simulink library "acc"  (R2021b)
settings: Solver=VariableStepAuto  StartTime=0.0  StopTime=10.0  RelTol=1e-3
undefined symbols (not defined in the file or in its folder): AACC_EHPSSpdCtrlMode_X_enum, AACC_EHPSSpdCtrlMode_Y_rad, ENUM__SASCALED_CALED, ENUM_BRAKEPEDAL_RELEASED, ENUM_CACENABLESTS_RUN, ENUM_DCDCENABLESTS_RUN, ENUM_EHPSCTRLMODE_FULLPWR, ENUM_EHPSCTRLMODE_NORMAL, ENUM_EHPSCTRLMODE_STEP1, ENUM_EHPSCTRLMODE_ZERO, ENUM_EHPSENABLESTS_INITIAL, ENUM_EHPSENABLESTS_READY, ENUM_EHPSENABLESTS_RUN, ENUM_PMMMODE_DRIVE, ENUM_PMMMODE_POWERUP, ENUM_TARGETGEAR_NEUTRAL, FALSE, KACC_AirPressInvalid_kpa, KACC_CACEnableFailTime_s, KACC_CACOverrunRcvTime_s, KACC_CACOverrunTime_min, KACC_CACOverTempDelayTime_s, KACC_CACOverTempRcv_s, KACC_CACPresLow_kPa, KACC_CACPressureSWRev_flg, KACC_CACPresWarn_kPa, KACC_CACPresWarn_ovrdflg_flg, KACC_CACPresWarn_ovrdval_flg, KACC_CACStopTime_s, KACC_CACTemp_C, KACC_CACTempRev_C, KACC_CACTempStop_C, KACC_CACTempWarn_C, KACC_CACValid_flg, KACC_CP2VAutoTracH_enum, KACC_CP2VDamStiffReqFA_pct, KACC_CP2VDamStiffReqLA_pct, KACC_CP2VDamStiffReqRA_pct, KACC_CP2VKneeCtrlMReq_enum, KACC_CP2VKneeReqFA_enum, KACC_CP2VKneeReqRA_enum, KACC_CP2VKneeReqRSide_enum, KACC_CP2VLA1PosCmd_enum, KACC_CP2VLA2PosCmd_enum, KACC_CP2VLvCtrlModeReq_enum, KACC_CP2VNLvReqFA_enum, KACC_CP2VNLvReqRA_enum, KACC_DCDCErrLvHoldtime_s, KACC_DTCACCReset_flg, KACC_DTCCACOverrun_cnt, KACC_EACErrLvHoldtime_s, KACC_ECASKneeSideSW_flg, KACC_EcasSw1Down_flg, KACC_EcasSw1Up_flg, KACC_EcasSw2M2_flg, KACC_EcasSw2Stop_flg, KACC_EcasSw3Knee_flg, KACC_EcasSw3M1_flg, KACC_EcasSwDebounceTime_s, KACC_ECASSwitch_flg ... (+30)
libraries: hcu_lib x20, simulink x3
(part 1 of 3)
settings Model: Creator=zack  LastModifiedBy=zack

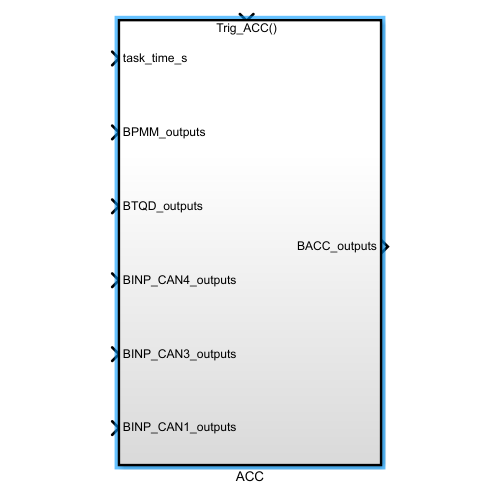
[thumbnail: Simulink's stored preview of the top-level diagram]
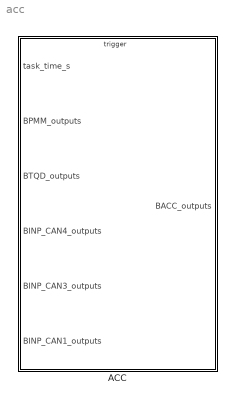
== system acc ==
  ACC : Subsystem  TreatAsAtomicUnit=on
      settings: RTWSystemCode=Nonreusable function  RTWFcnNameOpts=Use subsystem name  RTWFileNameOpts=Use subsystem name

== system acc/ACC ==
  task_time_s : Inport
  BPMM_outputs : Inport  Port=2  OutDataTypeStr=Bus: BPMM_outputs
  BTQD_outputs : Inport  Port=3  OutDataTypeStr=Bus: BTQD_outputs
  BINP_CAN4_outputs : Inport  Port=4  OutDataTypeStr=Bus: BINP_CAN4_outputs
  BINP_CAN3_outputs : Inport  Port=5  OutDataTypeStr=Bus: BINP_CAN3_outputs
  BINP_CAN1_outputs : Inport  Port=6  OutDataTypeStr=Bus: BINP_CAN1_outputs
  Trig_ACC : TriggerPort  TriggerType=function-call  VariantControl=(inherit)
  Input_Convert : Subsystem
  Main : Subsystem
  Model Info1 : hcu_lib/Model Info1  BlockCM=None  Frame=on  DisplayStringWithTags=|  HorizontalTextAlignment=Left  LeftAlignmentValue=0.02  SourceBlockDiagram=hcu_lib  TagMaxNumber=20
      | Model Version        : %<ModelVersion>
      | Creator                   : %<Creator>
      | Last Modified By    : %<LastModifiedBy>
      settings: SourceProductName=HCU Relative Block Library
  OutpConvert : Subsystem
  SCP_In : Subsystem
  SCP_Out : Subsystem
  BACC_outputs : Outport  OutDataTypeStr=Bus: BACC_outputs  VectorParamsAs1DForOutWhenUnconnected=off
  wires:
  task_time_s/1 -> SCP_In/1(task_time_s)
  BINP_CAN4_outputs/1 -> SCP_In/2(BINP_CAN4_outputs)
  BINP_CAN3_outputs/1 -> SCP_In/3(BINP_CAN3_outputs)
  BINP_CAN1_outputs/1 -> SCP_In/4(BINP_CAN1_outputs)
  BTQD_outputs/1 -> SCP_In/5(BTQD_outputs)
  BPMM_outputs/1 -> SCP_In/6(BPMM_outputs)
  SCP_In/1(BSCP_In_outputs) -> [BSCP_In_outputs]
  [BSCP_In_outputs] -> Input_Convert/1(BSCP_In_outputs)
  Input_Convert/1(BInpConvert_outputs) -> [BInpConvert_outputs]
  [BInpConvert_outputs] -> Main/2(BInpConvert_outputs)
  [BSCP_In_outputs] -> Main/1(BSCP_In_outputs)
  Main/1(BMain_outputs) -> [BMain_outputs]
  [BMain_outputs] -> Input_Convert/2(BMain_outputs)
  [BInpConvert_outputs] -> OutpConvert/2(BInpConvert_outputs)
  [BMain_outputs] -> OutpConvert/3(BMain_outputs)
  [BSCP_In_outputs] -> OutpConvert/1(BSCP_In_outputs)
  OutpConvert/1(BOutpConvert_outputs) -> [BOutpConvert_outputs]
  [BInpConvert_outputs] -> SCP_Out/1(BInpConvert_outputs)
  [BMain_outputs] -> SCP_Out/2(BMain_outputs)
  [BOutpConvert_outputs] -> SCP_Out/3(BOutpConvert_outputs)
  SCP_Out/1(BACC_outputs) -> BACC_outputs/1

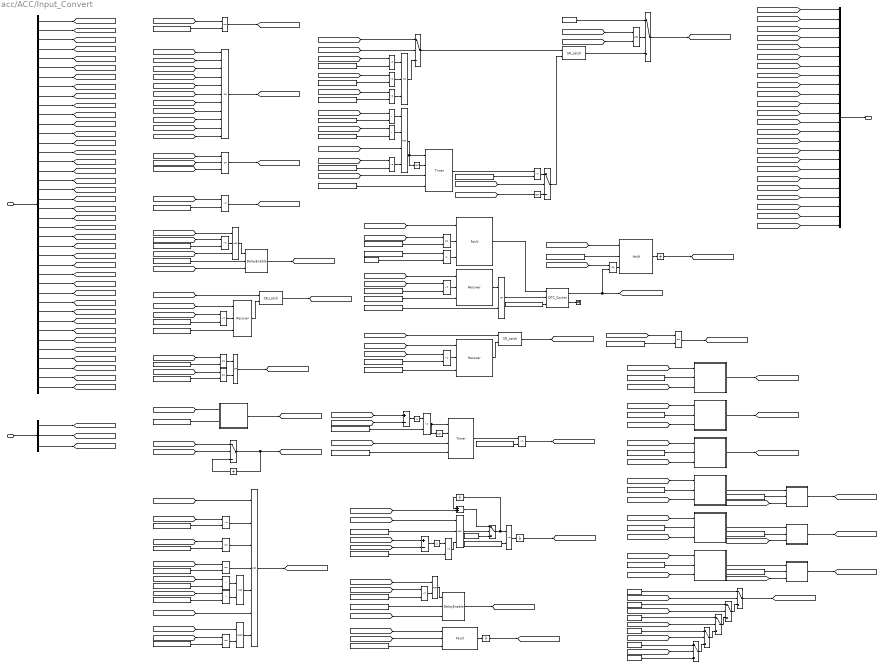
== system acc/ACC/Input_Convert ==
  note: ECAS Demand Determination From Pin
  note: EHPS Force Stop Detection
  note: EHPS Motor Speed Demand TimeOut Detection
  note: EHPS Disable Judgement
  note: Steering Wheel Moving Detection
  note: Steering Angle has been calabrated flag
  note: EHPS Error Hold Disable Judgment
  note: EHPS Cooling Mode Judgment
  note: Brake Pedal Released Flag
  note: EAC Pressure Sensor DDM
  note: EAC Pressure Switch DDM
  note: EAC Over Temperature Judgment
  note: EAC Pressure Low Judgment
  note: EAC Running Fail Judgment
  note: EAC Forece Stop Judgment
  note: EAC Error Hold Disable Judgment
  BSCP_In_outputs : Inport
  BMain_outputs : Inport  Port=2
  " EcasSw1Down Debounce" : Subsystem
  " EcasSw1Up Debounce" : Subsystem
  " EcasSw2Stop Debounce" : Subsystem
  AND : Logic  Inputs=4  AllPortsSameDT=off  OutDataTypeStr=boolean
  AND1 : Logic  AllPortsSameDT=off  OutDataTypeStr=boolean
  AND2 : Logic  AllPortsSameDT=off  OutDataTypeStr=boolean
  AND3 : Logic  Inputs=3  AllPortsSameDT=off  OutDataTypeStr=boolean
  AND5 : Logic  Operator=NAND  AllPortsSameDT=off  OutDataTypeStr=boolean
  Abs : Abs
  Abs1 : Abs
  Add : Sum  Inputs=+-
  Add1 : Sum  Inputs=+-
  Add2 : Sum
  Bus Creator : BusCreator  Inputs=24
  Bus Selector : BusSelector  OutputSignals=VINP_EBSBrakeSw_enum,VDMM_DTCFCShortBatt_flg,VDMM_DTCPCShortBatt_flg,VDMM_DTCRCShortBatt_flg,VDMM_DTCFCOpenGND_flg,VDMM_DTCPCOpenGND_flg,VDMM_DTCRCOpenGND_flg,VDMM_DTCFCStuckHigh_flg,VDMM_DTCRCStuckHigh_flg,VDMM_DTCFCStuckLow_flg,VDMM_DTCPCStuckLow_flg,VDMM_DTCRCStuckLow_flg,VDMM_DTCAirSwError_flg,VDMM_DTCAirSwStuckClose_flg,VDMM_DTCAirSwStuckOpen_flg,VINP_CACTemp_C,VINP_FDCCHASSISVCUEACPressSta_flg,VINP_AirPressureRC1_kPa,VINP_AirPressureFC2_kPa,VINP_AirPressurePC3_kPa,task_time_s,VINP_EACEnSta_enum,VPMM_EACEnableCompleted_flg,VDMM_DTCEACErrLv_flg,VPMM_SysPowerMode_enum,VDMM_DTCEHPSErrLv_flg,VINP_EHPSEnSta_enum,VINP_SASCaled_enum,VINP_StrWhlAng_rad,VINP_ParkBrakeSW_enum,VTQD_VCUVehSpd_kph,VINP_TransReqGear_enum,VDMM_DTCEHPSRlyNoFB_flg,VINP_EHPSMotorSpdSta_rpm,VINP_EcasSw1Up_flg,VINP_EcasSw1Down_flg,VINP_EcasSw2Stop_flg,VINP_EcasSw2M2_flg,VINP_EcasSw3M1_flg,VINP_EcasSw3Knee_flg
  Bus Selector1 : BusSelector  OutputSignals=VACC_CACEnableDem_flg,VACC_InitEHPSEnDem_flg,VACC_EHPSMotorDemSpd_rpm
  Constant : Constant  Value=ENUM_BRAKEPEDAL_RELEASED
  Constant1 : Constant  Value=KACC_CACPresLow_kPa
  Constant10 : Constant  Value=KACC_CACPresWarn_kPa
  Constant11 : Constant  Value=MIN2SEC
  Constant12 : Constant  Value=KACC_DTCCACOverrun_cnt
  Constant13 : Constant  Value=KACC_CACOverrunRcvTime_s
  Constant131 : Constant  Value=KACC_SpeedOverEHPSEnDemend_kph
  Constant{14..15,17,22} (4 alike) : Constant  Value=ENUM_CACENABLESTS_RUN
  Constant16 : Constant  Value=KACC_DTCACCReset_flg
  Constant18 : Constant  Value=KACC_CACEnableFailTime_s
  Constant19 : Constant  Value=KACC_CACOverrunTime_min
  Constant2 : Constant  Value=TRUE
  Constant20 : Constant  Value=KACC_CACStopTime_s
  Constant21 : Constant  Value=KACC_EACErrLvHoldtime_s
  Constant23 : Constant  Value=ENUM_PMMMODE_DRIVE  SampleTime=-1
  Constant24 : Constant  Value=ENUM_PMMMODE_POWERUP  SampleTime=-1
  Constant25 : Constant  Value=KACC_EHPSErrLvHoldtime_s
  Constant26 : Constant  Value=ENUM_EHPSENABLESTS_RUN
  Constant27 : Constant  Value=ENUM__SASCALED_CALED
  Constant28 : Constant  Value=KACC_StrWhlAngSampleTime_s
  Constant29 : Constant  Value=KACC_EHPSDisStrWhlDiv_rad
  Constant3 : Constant  Value=KACC_CACPresWarn_kPa
  Constant30 : Constant  Value=KACC_StrWhlNotMovingTime_s  OutDataTypeStr=single
  Constant31 : Constant  Value=KACC_StrWhlNotMovingTime_s  OutDataTypeStr=single
  Constant32 : Constant  Value=KACC_EHPSDisStrWhlHi_rad
  Constant33 : Constant  Value=KACC_EHPSDisStrWhlLo_rad
  Constant34 : Constant  Value=ENUM_PMMMODE_DRIVE
  Constant35 : Constant  Value=ENUM_TARGETGEAR_NEUTRAL
  Constant36 : Constant  Value=ENUM__SASCALED_CALED
  Constant37 : Constant  Value=KACC_EHPSCtrlModeStep2_flg
  Constant38 : Constant  Value=KACC_EHPSSpdDiv_rpm
  Constant39 : Constant  Value=ENUM_EHPSENABLESTS_RUN
  Constant4 : Constant  Value=KACC_CACPresWarn_kPa
  Constant40 : Constant  Value=KACC_EHPSEnableFailTime_s
  Constant41 : Constant  Value=KACC_EHPSStopTime_s
  Constant{42..47} (6 alike) : Constant  Value=KACC_EcasSwDebounceTime_s
  Constant48 : Constant  Value=KACC_EcasSwTrigHoldTime_s
  Constant49 : Constant  Value=KACC_EcasSwTrigHoldTime_s
  Constant5 : Constant  Value=KACC_SwitchFailSensorRef_kpa
  Constant50 : Constant  Value=KACC_EcasSwTrigHoldTime_s
  Constant51 : Constant  Value=uint8(0)
  Constant52 : Constant  Value=uint8(7)
  Constant53 : Constant  Value=uint8(2)
  Constant54 : Constant  Value=uint8(6)
  Constant55 : Constant  Value=uint8(1)
  Constant56 : Constant  Value=uint8(8)
  Constant6 : Constant  Value=KACC_SwitchFailSensorRef_kpa
  Constant62 : Constant  Value=ZERO_FLOAT
  Constant63 : Constant  Value=KACC_EHPSSpdDemTimeout_s
  Constant7 : Constant  Value=KACC_SwitchFailSensorRefRcv_s
  Constant8 : Constant  Value=KACC_SwitchFailSensorRefRcv_s
  Constant9 : Constant  Value=KACC_CACTempStop_C
  DTC_Couter : hcu_lib/Basic_Blocks/DTC_Couter
      settings: SourceProductName=HCU Relative Block Library
  DelayEnable : hcu_lib/Basic_Blocks/DelayEnable
      settings: SourceProductName=HCU Relative Block Library
  DelayEnable1 : hcu_lib/Basic_Blocks/DelayEnable
      settings: SourceProductName=HCU Relative Block Library
  EcasSw2M2 Debounce : Subsystem
  EcasSw3Knee Debounce : Subsystem
  EcasSw3M1 Debounce : Subsystem
  Equal{,1..2,5,9} (5 alike) : RelationalOperator  Operator===  OutDataTypeStr=boolean  RndMeth=Simplest
  Equal3 : RelationalOperator  Operator=<  OutDataTypeStr=boolean  RndMeth=Simplest
  Equal4 : RelationalOperator  Operator=<=  OutDataTypeStr=boolean  RndMeth=Simplest
  Equal6 : RelationalOperator  Operator=>  OutDataTypeStr=boolean  RndMeth=Simplest
  Fault : hcu_lib/Basic_Blocks/Fault  SystemSampleTime=-1  VariantActivationTime=update diagram  Latency=0  AutoFrameSizeCalculation=off
      settings: SourceProductName=HCU Relative Block Library
  Fault1 : hcu_lib/Basic_Blocks/Fault  SystemSampleTime=-1  VariantActivationTime=update diagram  Latency=0  AutoFrameSizeCalculation=off
      settings: SourceProductName=HCU Relative Block Library
  Hold1 : hcu_lib/Basic_Blocks/Hold  SystemSampleTime=-1  VariantActivationTime=update diagram  Latency=0  AutoFrameSizeCalculation=off
      settings: SourceProductName=HCU Relative Block Library
  Logical Operator : Logic  Operator=OR  AllPortsSameDT=off  OutDataTypeStr=boolean
  Logical Operator1 : Logic  AllPortsSameDT=off  OutDataTypeStr=boolean
  Logical Operator10 : Logic  Operator=OR  Inputs=3  AllPortsSameDT=off  OutDataTypeStr=boolean
  Logical Operator4 : Logic  Inputs=7  AllPortsSameDT=off  OutDataTypeStr=boolean
  Logical Operator5 : Logic  Inputs=3  AllPortsSameDT=off  OutDataTypeStr=boolean
  Logical Operator6 : Logic  Operator=OR  AllPortsSameDT=off  OutDataTypeStr=boolean
  NOT : Logic  Operator=NOT  AllPortsSameDT=off  OutDataTypeStr=boolean
  NOT1 : Logic  Operator=NOT  AllPortsSameDT=off  OutDataTypeStr=boolean
  NOT4 : Logic  Operator=NOT  AllPortsSameDT=off  OutDataTypeStr=boolean
  OR : Logic  Operator=OR  Inputs=11  AllPortsSameDT=off  OutDataTypeStr=boolean
  OR1 : Logic  Operator=OR  Inputs=3  AllPortsSameDT=off  OutDataTypeStr=boolean
  OR2 : Logic  Operator=OR  AllPortsSameDT=off  OutDataTypeStr=boolean
  Product : Product
  Recover : hcu_lib/Basic_Blocks/Recover  SystemSampleTime=-1  VariantActivationTime=update diagram  Latency=0  AutoFrameSizeCalculation=off
      settings: SourceProductName=HCU Relative Block Library
  Recover1 : hcu_lib/Basic_Blocks/Recover  SystemSampleTime=-1  VariantActivationTime=update diagram  Latency=0  AutoFrameSizeCalculation=off
      settings: SourceProductName=HCU Relative Block Library
  Recover2 : hcu_lib/Basic_Blocks/Recover  SystemSampleTime=-1  VariantActivationTime=update diagram  Latency=0  AutoFrameSizeCalculation=off
      settings: SourceProductName=HCU Relative Block Library
  Relational Operator{,8,11..12,16,18} (6 alike) : RelationalOperator  OutDataTypeStr=boolean  RndMeth=Simplest
  Relational Operator{1..2,9,15,19} (5 alike) : RelationalOperator  Operator=~=  OutDataTypeStr=boolean  RndMeth=Simplest
  Relational Operator10 : RelationalOperator  Operator===  OutDataTypeStr=boolean  RndMeth=Nearest
  Relational Operator{6..7,13,17} (4 alike) : RelationalOperator  Operator=<=  OutDataTypeStr=boolean  RndMeth=Simplest
  Relational Operator14 : RelationalOperator  Operator===  OutDataTypeStr=boolean  RndMeth=Nearest
  Relational Operator3 : RelationalOperator  Operator=>  OutDataTypeStr=boolean  RndMeth=Simplest
  Relational Operator4 : RelationalOperator  Operator===  OutDataTypeStr=boolean  RndMeth=Simplest
  Relational Operator5 : RelationalOperator  Operator=>  OutDataTypeStr=boolean  RndMeth=Simplest
  SR_Latch : hcu_lib/Basic_Blocks/SR_Latch
      settings: SourceProductName=HCU Relative Block Library
  SR_Latch1 : hcu_lib/Basic_Blocks/SR_Latch
      settings: SourceProductName=HCU Relative Block Library
  SR_Latch2 : hcu_lib/Basic_Blocks/SR_Latch
      settings: SourceProductName=HCU Relative Block Library
  Switch{,1..9} (10 alike) : Switch  Criteria=u2 ~= 0
      settings: AttributesFormatString=%<Criteria>
  Switch hold : Subsystem
  Switch hold1 : Subsystem
  Switch hold3 : Subsystem
  Terminator1 : Terminator
  Timer : hcu_lib/Basic_Blocks/Timer
      settings: SourceProductName=HCU Relative Block Library
  Timer1 : hcu_lib/Basic_Blocks/Timer
      settings: SourceProductName=HCU Relative Block Library
  Trigger : Subsystem  AncestorBlock=hcu_lib/Basic_Blocks/Fault
  Unit Delay{,1,3,5} (4 alike) : UnitDelay  InitialCondition=boolean(0)  SampleTime=-1  HasFrameUpgradeWarning=on
      settings: AttributesFormatString=%<InitialCondition>
  Unit Delay2 : UnitDelay  InitialCondition=single(0)  SampleTime=-1  HasFrameUpgradeWarning=on
      settings: AttributesFormatString=%<InitialCondition>
  BInpConvert_outputs : Outport
  wires:
  Constant24/1 -> Relational Operator14/2
  Logical Operator/1 -> [VACC_CoolingMode_flg]  "VACC_CoolingMode_flg"
  Relational Operator10/1 -> Logical Operator/2
  Constant23/1 -> Relational Operator10/2
  Relational Operator14/1 -> Logical Operator/1
  [VPMM_SysPowerMode_enum] -> Relational Operator10/1
  [VPMM_SysPowerMode_enum] -> Relational Operator14/1
  Bus Selector/24 -> [VDMM_DTCEACErrLv_flg]  "<VDMM_DTCEACErrLv_flg>"
  [VDMM_DTCEACErrLv_flg] -> SR_Latch/1
  [VINP_EACEnSta_enum] -> Relational Operator9/1
  [task_time_s] -> Recover1/1
  Relational Operator9/1 -> Recover1/2
  Constant21/1 -> Recover1/3
  Recover1/1 -> SR_Latch/2
  Constant22/1 -> Relational Operator9/2
  SR_Latch/1 -> [VACC_EACErrLvHoldDis_flg]  "VACC_EACErrLvHoldDis_flg"
  Constant20/1 -> Hold1/2
  [VACC_CACRunFail_flg] -> Logical Operator6/1
  Constant19/1 -> Product/1
  Bus Selector/23 -> [VPMM_EACEnableCompleted_flg]  "<VPMM_EACEnableCompleted_flg>"
  Bus Selector/22 -> [VINP_EACEnSta_enum]  "<VINP_EACEnSta_enum>"
  Constant18/1 -> DelayEnable/2
  DelayEnable/1 -> [VACC_CACRunFail_flg]  "VACC_CACRunFail_flg"
  [VACC_CACEnableDem_flg] -> Logical Operator5/3
  Relational Operator1/1 -> Logical Operator5/2
  [task_time_s] -> DelayEnable/3
  Constant14/1 -> Relational Operator2/2
  Logical Operator6/1 -> Hold1/3
  Constant15/1 -> Relational Operator1/2
  Product/1 -> Fault/3
  [VINP_EACEnSta_enum] -> Relational Operator1/1
  Logical Operator5/1 -> DelayEnable/1
  [task_time_s] -> Fault/1
  Constant17/1 -> Relational Operator4/2
  Constant11/1 -> Product/2
  Relational Operator4/1 -> Fault/2
  OR2/1 -> DTC_Couter/2
  Hold1/1 -> Unit Delay/1
  Unit Delay/1 -> [VACC_CACForceStop_flg]  "VACC_CACForceStop_flg"
  [VINP_EACEnSta_enum] -> Relational Operator4/1
  DTC_Couter/1 -> [VACC_CACOverrun_flg], Logical Operator6/2  "VACC_CACOverrun_flg"
  [task_time_s] -> Hold1/1
  DTC_Couter/2 -> Terminator1/1
  Constant12/1 -> DTC_Couter/3
  Relational Operator2/1 -> Recover/2
  [VINP_EACEnSta_enum] -> Relational Operator2/1
  Recover/1 -> OR2/1
  [task_time_s] -> Recover/1
  Constant13/1 -> Recover/3
  [VPMM_EACEnableCompleted_flg] -> Logical Operator5/1
  Fault/1 -> DTC_Couter/1
  Constant16/1 -> OR2/2
  Bus Selector/21 -> [task_time_s]  "<task_time_s>"
  Bus Selector/20 -> [VINP_AirPressurePC3_kPa]  "<VINP_AirPressurePC3_kPa>"
  Bus Selector/19 -> [VINP_AirPressureFC2_kPa]  "<VINP_AirPressureFC2_kPa>"
  Bus Selector/18 -> [VINP_AirPressureRC1_kPa]  "<VINP_AirPressureRC1_kPa>"
  Bus Selector/17 -> [VINP_FDCCHASSISVCUEACPressSta_flg]  "<VINP_FDCCHASSISVCUEACPressSta_flg>"
  Constant10/1 -> Relational Operator7/2
  Constant4/1 -> Relational Operator6/2
  Constant3/1 -> Relational Operator13/2
  Switch4/1 -> [VACC_CACPresLow_flg]  "VACC_CACPresLow_flg"
  Relational Operator7/1 -> Logical Operator10/1
  [VACC_EACRefSwitchEnable_flg] -> Switch3/2
  [VINP_AirPressureFC2_kPa] -> Relational Operator7/1
  [VINP_AirPressureRC1_kPa] -> Relational Operator6/1
  [VACC_EACRefSensorDis_flg] -> AND/3
  [VINP_FDCCHASSISVCUEACPressSta_flg] -> NOT/1
  [VINP_AirPressureFC2_kPa] -> Relational Operator3/1
  [VINP_FDCCHASSISVCUEACPressSta_flg] -> Switch3/1
  [VACC_EACRefSensorDis_flg] -> AND1/2
  Relational Operator11/1 -> AND/4
  Constant2/1 -> Switch4/1
  [VINP_AirPressurePC3_kPa] -> Relational Operator13/1
  Constant7/1 -> Timer/4
  Constant6/1 -> Relational Operator5/2
  Timer/1 -> Relational Operator8/1
  AND/1 -> NOT1/1, Timer/1
  Relational Operator8/1 -> Switch2/1
  Constant5/1 -> Relational Operator3/2
  Relational Operator3/1 -> AND/1
  Constant8/1 -> Relational Operator8/2
  [VINP_AirPressurePC3_kPa] -> Relational Operator11/1
  Constant1/1 -> Relational Operator11/2
  [VINP_AirPressureRC1_kPa] -> Relational Operator5/1
  Relational Operator6/1 -> Logical Operator10/2
  Switch3/1 -> SR_Latch1/1
  [VACC_EACRefSensorDis_flg] -> Switch2/2
  Logical Operator10/1 -> Switch3/3  "VACC_EACSensorPresLow_flg"
  Relational Operator13/1 -> Logical Operator10/3
  [VACC_EACRefSwitchEnable_flg] -> AND1/1
  Switch2/1 -> SR_Latch1/2  "VACC_EACPresLowReset_flg"
  SR_Latch1/1 -> Switch4/3
  AND1/1 -> Switch4/2
  NOT1/1 -> Timer/2
  NOT/1 -> Switch2/3
  [task_time_s] -> Timer/3
  Relational Operator5/1 -> AND/2
  Bus Selector/16 -> [VINP_CACTemp_C]  "<VINP_CACTemp_C>"
  Relational Operator12/1 -> [VACC_CACOverTempStop_flg]  "VACC_CACOverTempStop_flg"
  Constant9/1 -> Relational Operator12/2
  [VINP_CACTemp_C] -> Relational Operator12/1
  Bus Selector/15 -> [VDMM_DTCAirSwStuckOpen_flg]  "<VDMM_DTCAirSwStuckOpen_flg>"
  Bus Selector/14 -> [VDMM_DTCAirSwStuckClose_flg]  "<VDMM_DTCAirSwStuckClose_flg>"
  Bus Selector/13 -> [VDMM_DTCAirSwError_flg]  "<VDMM_DTCAirSwError_flg>"
  [VDMM_DTCAirSwStuckClose_flg] -> OR1/2
  OR1/1 -> [VACC_EACRefSensorDis_flg]  "VACC_EACRefSensorDis_flg"
  [VDMM_DTCAirSwStuckOpen_flg] -> OR1/3
  [VDMM_DTCAirSwError_flg] -> OR1/1
  [VDMM_DTCFCOpenGND_flg] -> OR/4
  [VDMM_DTCPCShortBatt_flg] -> OR/2
  [VDMM_DTCFCStuckLow_flg] -> OR/9
  [VDMM_DTCPCOpenGND_flg] -> OR/5
  [VDMM_DTCFCShortBatt_flg] -> OR/1
  [VDMM_DTCPCStuckLow_flg] -> OR/10
  [VDMM_DTCFCStuckHigh_flg] -> OR/7
  [VDMM_DTCRCStuckLow_flg] -> OR/11
  [VDMM_DTCRCStuckHigh_flg] -> OR/8
  OR/1 -> [VACC_EACRefSwitchEnable_flg]  "VACC_EACRefSwitchEnable_flg"
  [VDMM_DTCRCOpenGND_flg] -> OR/6
  [VDMM_DTCRCShortBatt_flg] -> OR/3
  Bus Selector/12 -> [VDMM_DTCRCStuckLow_flg]  "<VDMM_DTCRCStuckLow_flg>"
  Bus Selector/11 -> [VDMM_DTCPCStuckLow_flg]  "<VDMM_DTCPCStuckLow_flg>"
  Bus Selector/10 -> [VDMM_DTCFCStuckLow_flg]  "<VDMM_DTCFCStuckLow_flg>"
  Bus Selector/9 -> [VDMM_DTCRCStuckHigh_flg]  "<VDMM_DTCRCStuckHigh_flg>"
  Bus Selector/8 -> [VDMM_DTCFCStuckHigh_flg]  "<VDMM_DTCFCStuckHigh_flg>"
  Bus Selector/7 -> [VDMM_DTCRCOpenGND_flg]  "<VDMM_DTCRCOpenGND_flg>"
  Bus Selector/6 -> [VDMM_DTCPCOpenGND_flg]  "<VDMM_DTCPCOpenGND_flg>"
  Bus Selector/5 -> [VDMM_DTCFCOpenGND_flg]  "<VDMM_DTCFCOpenGND_flg>"
  Bus Selector/4 -> [VDMM_DTCRCShortBatt_flg]  "<VDMM_DTCRCShortBatt_flg>"
  Bus Selector/3 -> [VDMM_DTCPCShortBatt_flg]  "<VDMM_DTCPCShortBatt_flg>"
  Bus Selector/2 -> [VDMM_DTCFCShortBatt_flg]  "<VDMM_DTCFCShortBatt_flg>"
  Equal/1 -> [VACC_EBSBrakeRelease_flg]  "VACC_EBSBrakeRelease_flg"
  Constant/1 -> Equal/2
  [VINP_EBSBrakeSw_enum] -> Equal/1
  Bus Selector/1 -> [VINP_EBSBrakeSw_enum]  "<VINP_EBSBrakeSw_enum>"
  BSCP_In_outputs/1 -> Bus Selector/1
  Bus Selector/25 -> [VPMM_SysPowerMode_enum]  "<VPMM_SysPowerMode_enum>"
  Relational Operator15/1 -> Recover2/2
  Recover2/1 -> SR_Latch2/2
  [VINP_EHPSEnSta_enum] -> Relational Operator15/1
  [VDMM_DTCEHPSErrLv_flg] -> SR_Latch2/1
  [task_time_s] -> Recover2/1
  Constant25/1 -> Recover2/3
  SR_Latch2/1 -> [VACC_EHPSErrLvHoldDis_flg]  "VACC_EHPSErrLvHoldDis_flg"
  Constant26/1 -> Relational Operator15/2
  Bus Selector/26 -> [VDMM_DTCEHPSErrLv_flg]  "<VDMM_DTCEHPSErrLv_flg>"
  Bus Selector/27 -> [VINP_EHPSEnSta_enum]  "<VINP_EHPSEnSta_enum>"
  [VINP_SASCaled_enum] -> Equal5/1
  Constant27/1 -> Equal5/2
  Equal5/1 -> [VACC_SASCalFinish_flg]  "VACC_SASCalFinish_flg"
  Bus Selector/28 -> [VINP_SASCaled_enum]  "<VINP_SASCaled_enum>"
  [task_time_s] -> Trigger/1(task_time_s)
  Trigger/1(ActionFlag) -> [VACC_StrWhlAngMemDet_flg]  "VACC_StrWhlAngMemDet_flg"
  Constant28/1 -> Trigger/2(DectectTime)
  [VINP_StrWhlAng_rad] -> Switch1/1
  Switch1/1 -> Unit Delay1/1, [VACC_StrWhlAngLast_rad]  "VACC_StrWhlAngLast_rad"
  Unit Delay1/1 -> Switch1/3
  [VACC_StrWhlAngMemDet_flg] -> Switch1/2
  Bus Selector/29 -> [VINP_StrWhlAng_rad]  "<VINP_StrWhlAng_rad>"
  Relational Operator16/1 -> [VACC_StrWhlNotMoving_flg]  "VACC_StrWhlNotMoving_flg"
  Abs/1 -> Equal4/1
  Timer1/1 -> Relational Operator16/1
  Add/1 -> Abs/1
  [VACC_StrWhlAngLast_rad] -> Add/2
  Equal4/1 -> Timer1/1, NOT4/1
  [VINP_StrWhlAng_rad] -> Add/1
  [task_time_s] -> Timer1/3
  Constant29/1 -> Equal4/2
  NOT4/1 -> Timer1/2
  Constant31/1 -> Timer1/4
  Constant30/1 -> Relational Operator16/2
  [VINP_ParkBrakeSW_enum] -> Logical Operator4/1
  Constant34/1 -> Equal9/2
  [VPMM_SysPowerMode_enum] -> Equal9/1
  Constant36/1 -> Equal2/2
  AND5/1 -> Logical Operator4/7
  [VINP_SASCaled_enum] -> Equal2/1
  Constant33/1 -> Equal6/2
  Equal6/1 -> AND2/2
  [VINP_StrWhlAng_rad] -> Equal6/1
  Constant32/1 -> Equal3/2
  Relational Operator17/1 -> Logical Operator4/2
  Constant131/1 -> Relational Operator17/2
  Constant35/1 -> Equal1/2
  Equal2/1 -> Logical Operator4/4
  [VINP_StrWhlAng_rad] -> Equal3/1
  Equal3/1 -> AND2/1
  Equal1/1 -> Logical Operator4/3
  [VACC_StrWhlNotMoving_flg] -> Logical Operator4/6
  Logical Operator4/1 -> [VACC_EHPSDisable_flg]  "VACC_EHPSDisable_flg"
  Equal9/1 -> AND5/2
  AND2/1 -> Logical Operator4/5
  [VINP_TransReqGear_enum] -> Equal1/1
  [VTQD_VCUVehSpd_kph] -> Relational Operator17/1
  [VDMM_DTCEHPSRlyNoFB_flg] -> AND5/1
  Bus Selector/30 -> [VINP_ParkBrakeSW_enum]  "<VINP_ParkBrakeSW_enum>"
  Bus Selector/31 -> [VTQD_VCUVehSpd_kph]  "<VTQD_VCUVehSpd_kph>"
  Bus Selector/32 -> [VINP_TransReqGear_enum]  "<VINP_TransReqGear_enum>"
  Bus Selector/33 -> [VDMM_DTCEHPSRlyNoFB_flg]  "<VDMM_DTCEHPSRlyNoFB_flg>"
  Constant37/1 -> AND3/2
  Add2/1 -> Switch6/1
  Relational Operator18/1 -> Unit Delay5/1
  Unit Delay5/1 -> [VACC_EHPSSpdDemTimeout_flg]  "VACC_EHPSSpdDemTimeout_flg"
  [VACC_InitEHPSEnDem_flg] -> AND3/1
  Constant62/1 -> Switch6/3
  Add1/1 -> Abs1/1
  Constant63/1 -> Relational Operator18/2
  AND3/1 -> Switch6/2
  [task_time_s] -> Add2/2
  Unit Delay2/1 -> Add2/1
  Relational Operator/1 -> AND3/3
  Abs1/1 -> Relational Operator/1
  [VINP_EHPSMotorSpdSta_rpm] -> Add1/2
  [VACC_EHPSMotorDemSpd_rpm] -> Add1/1
  Switch6/1 -> Unit Delay2/1, Relational Operator18/1
  Constant38/1 -> Relational Operator/2
  Bus Selector/34 -> [VINP_EHPSMotorSpdSta_rpm]  "<VINP_EHPSMotorSpdSta_rpm>"
  Fault1/1 -> Unit Delay3/1
  [task_time_s] -> Fault1/1
  [VACC_EHPSEnTimeout_flg] -> Fault1/2
  Logical Operator1/1 -> DelayEnable1/1
  DelayEnable1/1 -> [VACC_EHPSEnTimeout_flg]  "VACC_EHPSEnTimeout_flg"
  Constant41/1 -> Fault1/3
  [task_time_s] -> DelayEnable1/3
  Relational Operator19/1 -> Logical Operator1/2
  [VACC_InitEHPSEnDem_flg] -> Logical Operator1/1
  Constant40/1 -> DelayEnable1/2
  [VINP_EHPSEnSta_enum] -> Relational Operator19/1
  Unit Delay3/1 -> [VACC_EHPSForceStop_flg]  "VACC_EHPSForceStop_flg"
  Constant39/1 -> Relational Operator19/2
  [VACC_CACRunFail_flg] -> Bus Creator/5
  [VACC_CACOverTempStop_flg] -> Bus Creator/4
  [VACC_EACErrLvHoldDis_flg] -> Bus Creator/6
  [VACC_EACRefSensorDis_flg] -> Bus Creator/3
  [VACC_CoolingMode_flg] -> Bus Creator/7
  [VACC_EACRefSwitchEnable_flg] -> Bus Creator/2
  [VACC_StrWhlNotMoving_flg] -> Bus Creator/8
  [VACC_EBSBrakeRelease_flg] -> Bus Creator/1
  [VACC_EHPSDisable_flg] -> Bus Creator/9
  [VACC_EHPSSpdDemTimeout_flg] -> Bus Creator/10
  [VACC_EHPSForceStop_flg] -> Bus Creator/11
  [VACC_CACPresLow_flg] -> Bus Creator/12
  [VACC_CACForceStop_flg] -> Bus Creator/13
  [VACC_EHPSErrLvHoldDis_flg] -> Bus Creator/14
  [VACC_SASCalFinish_flg] -> Bus Creator/15
  Bus Creator/1 -> BInpConvert_outputs/1  "BInpConvert_outputs"
  BMain_outputs/1 -> Bus Selector1/1
  Bus Selector1/2 -> [VACC_InitEHPSEnDem_flg]  "<VACC_InitEHPSEnDem_flg>"
  Bus Selector1/3 -> [VACC_EHPSMotorDemSpd_rpm]  "<VACC_EHPSMotorDemSpd_rpm>"
  Bus Selector1/1 -> [VACC_CACEnableDem_flg]  "<VACC_CACEnableDem_flg>"
  [VACC_CACOverrun_flg] -> Bus Creator/16
  [VACC_EHPSEnTimeout_flg] -> Bus Creator/17
  Bus Selector/35 -> [VINP_EcasSw1Up_flg]  "<VINP_EcasSw1Up_flg>"
  Bus Selector/36 -> [VINP_EcasSw1Down_flg]  "<VINP_EcasSw1Down_flg>"
  Bus Selector/37 -> [VINP_EcasSw2Stop_flg]  "<VINP_EcasSw2Stop_flg>"
  Bus Selector/38 -> [VINP_EcasSw2M2_flg]  "<VINP_EcasSw2M2_flg>"
  Bus Selector/39 -> [VINP_EcasSw3M1_flg]  "<VINP_EcasSw3M1_flg>"
  Bus Selector/40 -> [VINP_EcasSw3Knee_flg]  "<VINP_EcasSw3Knee_flg>"
  [VINP_EcasSw1Up_flg] -> " EcasSw1Up Debounce"/1(signal_raw)
  Constant42/1 -> " EcasSw1Up Debounce"/2(time_limit)
  [task_time_s] -> " EcasSw1Up Debounce"/3(time_step)
  " EcasSw1Up Debounce"/1(signal_out) -> [VACC_EcasSw1Up_flg]  "VACC_EcasSw1Up_flg"
  " EcasSw1Down Debounce"/1(signal_out) -> [VACC_EcasSw1Down_flg]  "VACC_EcasSw1Down_flg"
  [task_time_s] -> " EcasSw1Down Debounce"/3(time_step)
  [VINP_EcasSw1Down_flg] -> " EcasSw1Down Debounce"/1(signal_raw)
  Constant43/1 -> " EcasSw1Down Debounce"/2(time_limit)
  Constant44/1 -> " EcasSw2Stop Debounce"/2(time_limit)
  [VINP_EcasSw2Stop_flg] -> " EcasSw2Stop Debounce"/1(signal_raw)
  [task_time_s] -> " EcasSw2Stop Debounce"/3(time_step)
  " EcasSw2Stop Debounce"/1(signal_out) -> [VACC_EcasSw2Stop_flg]  "VACC_EcasSw2Stop_flg"
  [task_time_s] -> EcasSw2M2 Debounce/3(time_step)
  [VINP_EcasSw2M2_flg] -> EcasSw2M2 Debounce/1(signal_raw)
  Constant45/1 -> EcasSw2M2 Debounce/2(time_limit)
  Constant46/1 -> EcasSw3M1 Debounce/2(time_limit)
  [VINP_EcasSw3M1_flg] -> EcasSw3M1 Debounce/1(signal_raw)
  [task_time_s] -> EcasSw3M1 Debounce/3(time_step)
  [task_time_s] -> EcasSw3Knee Debounce/3(time_step)
  [VINP_EcasSw3Knee_flg] -> EcasSw3Knee Debounce/1(signal_raw)
  Constant47/1 -> EcasSw3Knee Debounce/2(time_limit)
  EcasSw2M2 Debounce/1(signal_out) -> Switch hold/1(signal_in)
  [task_time_s] -> Switch hold/3(time_step)
  Constant48/1 -> Switch hold/2(hold_time)
  Constant49/1 -> Switch hold3/2(hold_time)
  [task_time_s] -> Switch hold3/3(time_step)
  EcasSw3M1 Debounce/1(signal_out) -> Switch hold3/1(signal_in)
  [task_time_s] -> Switch hold1/3(time_step)
  Constant50/1 -> Switch hold1/2(hold_time)
  EcasSw3Knee Debounce/1(signal_out) -> Switch hold1/1(signal_in)
  Switch hold1/1(signal_out) -> [VACC_EcasSw3Knee_flg]  "VACC_EcasSw3Knee_flg"
  Switch hold/1(signal_out) -> [VACC_EcasSw2M2_flg]  "VACC_EcasSw2M2_flg"
  Switch hold3/1(signal_out) -> [VACC_EcasSw3M1_flg]  "VACC_EcasSw3M1_flg"
  [VACC_EcasSw1Down_flg] -> Switch/2
  Constant51/1 -> Switch/3
  Constant52/1 -> Switch/1
  Constant54/1 -> Switch5/1
  [VACC_EcasSw1Up_flg] -> Switch5/2
  Switch/1 -> Switch5/3
  [VACC_EcasSw2M2_flg] -> Switch7/2
  Constant53/1 -> Switch7/1
  Switch5/1 -> Switch7/3
  Constant55/1 -> Switch8/1
  [VACC_EcasSw3M1_flg] -> Switch8/2
  Switch7/1 -> Switch8/3
  [VACC_EcasSw2Stop_flg] -> Switch9/2
  Constant56/1 -> Switch9/1
  Switch8/1 -> Switch9/3
  Switch9/1 -> [VACC_EcasNLvReq_enum]  "VACC_EcasNLvReq_enum"
  [VACC_EcasSw1Up_flg] -> Bus Creator/18
  [VACC_EcasSw1Down_flg] -> Bus Creator/19
  [VACC_EcasSw2Stop_flg] -> Bus Creator/20
  [VACC_EcasSw2M2_flg] -> Bus Creator/21
  [VACC_EcasSw3M1_flg] -> Bus Creator/22
  [VACC_EcasSw3Knee_flg] -> Bus Creator/23
  [VACC_EcasNLvReq_enum] -> Bus Creator/24

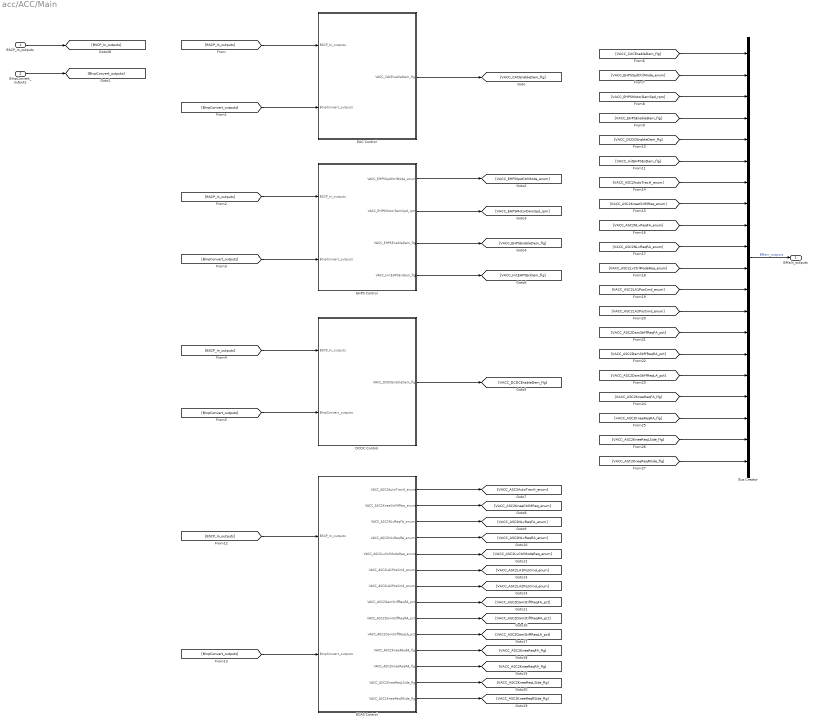
== system acc/ACC/Main ==
  BSCP_In_outputs : Inport
  BInpConvert_outputs : Inport  Port=2
  Bus Creator : BusCreator  Inputs=20
  DCDC Control : Subsystem
  EAC Control : Subsystem
  ECAS Control : Subsystem
  EHPS Control : Subsystem
  BMain_outputs : Outport
  wires:
  BSCP_In_outputs/1 -> [BSCP_In_outputs]
  BInpConvert_outputs/1 -> [BInpConvert_outputs]
  [BInpConvert_outputs] -> EAC Control/2(BInpConvert_outputs)
  [BSCP_In_outputs] -> EAC Control/1(BSCP_In_outputs)
  EAC Control/1(VACC_CACEnableDem_flg) -> [VACC_CACEnableDem_flg]
  [BSCP_In_outputs] -> EHPS Control/1(BSCP_In_outputs)
  [BInpConvert_outputs] -> EHPS Control/2(BInpConvert_outputs)
  EHPS Control/1(VACC_EHPSSpdCtrlMode_enum) -> [VACC_EHPSSpdCtrlMode_enum]
  EHPS Control/2(VACC_EHPSMotorDemSpd_rpm) -> [VACC_EHPSMotorDemSpd_rpm]
  EHPS Control/3(VACC_EHPSEnableDem_flg) -> [VACC_EHPSEnableDem_flg]
  [BSCP_In_outputs] -> DCDC Control/1(BSCP_In_outputs)
  [BInpConvert_outputs] -> DCDC Control/2(BInpConvert_outputs)
  DCDC Control/1(VACC_DCDCEnableDem_flg) -> [VACC_DCDCEnableDem_flg]
  [VACC_CACEnableDem_flg] -> Bus Creator/1
  [VACC_EHPSSpdCtrlMode_enum] -> Bus Creator/2
  [VACC_EHPSMotorDemSpd_rpm] -> Bus Creator/3
  [VACC_EHPSEnableDem_flg] -> Bus Creator/4
  [VACC_DCDCEnableDem_flg] -> Bus Creator/5
  Bus Creator/1 -> BMain_outputs/1  "BMain_outputs"
  EHPS Control/4(VACC_InitEHPSEnDem_flg) -> [VACC_InitEHPSEnDem_flg]
  [VACC_InitEHPSEnDem_flg] -> Bus Creator/6
  [BSCP_In_outputs] -> ECAS Control/1(BSCP_In_outputs)
  [BInpConvert_outputs] -> ECAS Control/2(BInpConvert_outputs)
  ECAS Control/1(VACC_ASC2AutoTracH_enum) -> [VACC_ASC2AutoTracH_enum]
  ECAS Control/2(VACC_ASC2KneeCtrlMReq_enum) -> [VACC_ASC2KneeCtrlMReq_enum]
  ECAS Control/3(VACC_ASC2NLvReqFA_enum) -> [VACC_ASC2NLvReqFA_enum]
  ECAS Control/4(VACC_ASC2NLvReqRA_enum) -> [VACC_ASC2NLvReqRA_enum]
  ECAS Control/5(VACC_ASC2LvCtrlModeReq_enum) -> [VACC_ASC2LvCtrlModeReq_enum]
  ECAS Control/6(VACC_ASC2LA1PosCmd_enum) -> [VACC_ASC2LA1PosCmd_enum]
  ECAS Control/7(VACC_ASC2LA2PosCmd_enum) -> [VACC_ASC2LA2PosCmd_enum]
  ECAS Control/8(VACC_ASC2DamStiffReqFA_pct) -> [VACC_ASC2DamStiffReqFA_pct]
  ECAS Control/9(VACC_ASC2DamStiffReqRA_pct) -> [VACC_ASC2DamStiffReqRA_pct]
  ECAS Control/10(VACC_ASC2DamStiffReqLA_pct) -> [VACC_ASC2DamStiffReqLA_pct]
  ECAS Control/11(VACC_ASC2KneeReqFA_flg) -> [VACC_ASC2KneeReqFA_flg]
  ECAS Control/12(VACC_ASC2KneeReqRA_flg) -> [VACC_ASC2KneeReqRA_flg]
  ECAS Control/13(VACC_ASC2KneeReqLSide_flg) -> [VACC_ASC2KneeReqLSide_flg]
  ECAS Control/14(VACC_ASC2KneeReqRSide_flg) -> [VACC_ASC2KneeReqRSide_flg]
  [VACC_ASC2AutoTracH_enum] -> Bus Creator/7
  [VACC_ASC2KneeCtrlMReq_enum] -> Bus Creator/8
  [VACC_ASC2NLvReqFA_enum] -> Bus Creator/9
  [VACC_ASC2NLvReqRA_enum] -> Bus Creator/10
  [VACC_ASC2LvCtrlModeReq_enum] -> Bus Creator/11
  [VACC_ASC2LA1PosCmd_enum] -> Bus Creator/12
  [VACC_ASC2LA2PosCmd_enum] -> Bus Creator/13
  [VACC_ASC2DamStiffReqFA_pct] -> Bus Creator/14
  [VACC_ASC2DamStiffReqRA_pct] -> Bus Creator/15
  [VACC_ASC2DamStiffReqLA_pct] -> Bus Creator/16
  [VACC_ASC2KneeReqFA_flg] -> Bus Creator/17
  [VACC_ASC2KneeReqRA_flg] -> Bus Creator/18
  [VACC_ASC2KneeReqLSide_flg] -> Bus Creator/19
  [VACC_ASC2KneeReqRSide_flg] -> Bus Creator/20

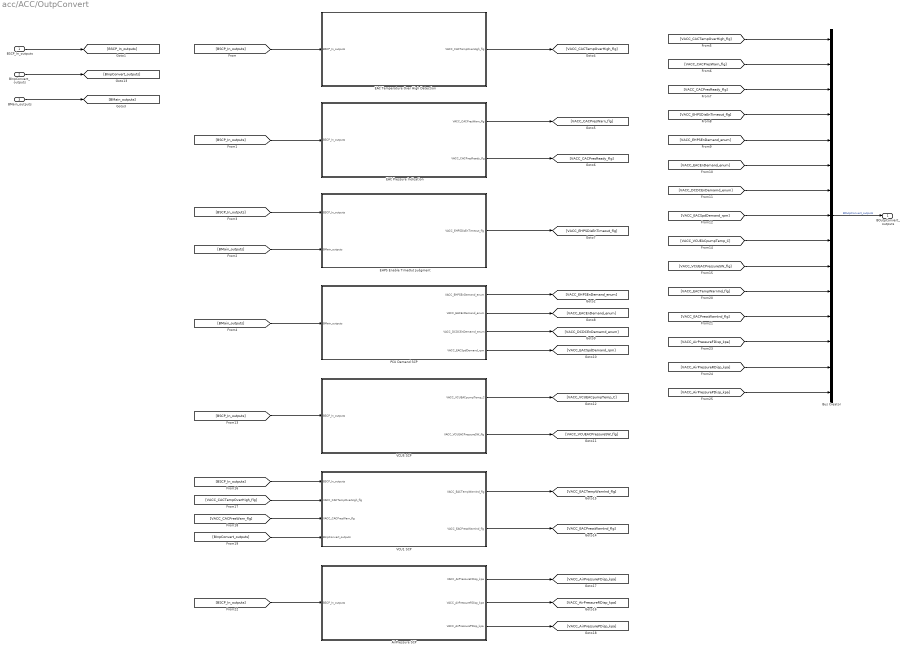
== system acc/ACC/OutpConvert ==
  BSCP_In_outputs : Inport
  BInpConvert_outputs : Inport  Port=2
  BMain_outputs : Inport  Port=3
  AirPressure SCP : Subsystem
  Bus Creator : BusCreator  Inputs=15
  EAC Pressure Indication : Subsystem
  EAC Temperature Over High Detection : Subsystem
  EHPS Enable TimeOut Judgment : Subsystem
  PCU Demand SCP : Subsystem
  VCU1 SCP : Subsystem
  VCU5 SCP : Subsystem
  BOutpConvert_outputs : Outport
  wires:
  BSCP_In_outputs/1 -> [BSCP_In_outputs]
  BInpConvert_outputs/1 -> [BInpConvert_outputs]
  BMain_outputs/1 -> [BMain_outputs]
  [BSCP_In_outputs] -> EAC Temperature Over High Detection/1(BSCP_In_outputs)
  EAC Temperature Over High Detection/1(VACC_CACTempOverHigh_flg) -> [VACC_CACTempOverHigh_flg]
  [BSCP_In_outputs] -> EAC Pressure Indication/1(BSCP_In_outputs)
  EAC Pressure Indication/1(VACC_CACPresWarn_flg) -> [VACC_CACPresWarn_flg]
  EAC Pressure Indication/2(VACC_CACPresReady_flg) -> [VACC_CACPresReady_flg]
  [BMain_outputs] -> EHPS Enable TimeOut Judgment/2(BMain_outputs)
  [BSCP_In_outputs] -> EHPS Enable TimeOut Judgment/1(BSCP_In_outputs)
  EHPS Enable TimeOut Judgment/1(VACC_EHPSDisEnTimeout_flg) -> [VACC_EHPSDisEnTimeout_flg]
  [BMain_outputs] -> PCU Demand SCP/1(BMain_outputs)
  PCU Demand SCP/1(VACC_EHPSEnDemand_enum) -> [VACC_EHPSEnDemand_enum]
  PCU Demand SCP/2(VACC_EACEnDemand_enum) -> [VACC_EACEnDemand_enum]
  PCU Demand SCP/3(VACC_DCDCEnDemamd_enum) -> [VACC_DCDCEnDemamd_enum]
  PCU Demand SCP/4(VACC_EACSpdDemand_rpm) -> [VACC_EACSpdDemand_rpm]
  [VACC_CACTempOverHigh_flg] -> Bus Creator/1
  [VACC_CACPresWarn_flg] -> Bus Creator/2
  [VACC_CACPresReady_flg] -> Bus Creator/3
  [VACC_EHPSDisEnTimeout_flg] -> Bus Creator/4
  [VACC_EHPSEnDemand_enum] -> Bus Creator/5
  [VACC_EACEnDemand_enum] -> Bus Creator/6
  [VACC_DCDCEnDemamd_enum] -> Bus Creator/7
  [VACC_EACSpdDemand_rpm] -> Bus Creator/8
  Bus Creator/1 -> BOutpConvert_outputs/1  "BOutpConvert_outputs"
  [BSCP_In_outputs] -> VCU5 SCP/1(BSCP_In_outputs)
  VCU5 SCP/1(VACC_VCUEACpumpTemp_C) -> [VACC_VCUEACpumpTemp_C]
  VCU5 SCP/2(VACC_VCUEACPressureSW_flg) -> [VACC_VCUEACPressureSW_flg]
  [VACC_VCUEACpumpTemp_C] -> Bus Creator/9
  [VACC_VCUEACPressureSW_flg] -> Bus Creator/10
  [BSCP_In_outputs] -> VCU1 SCP/1(BSCP_In_outputs)
  [VACC_CACTempOverHigh_flg] -> VCU1 SCP/2(VACC_CACTempOverHigh_flg)
  [VACC_CACPresWarn_flg] -> VCU1 SCP/3(VACC_CACPresWarn_flg)
  [BInpConvert_outputs] -> VCU1 SCP/4(BInpConvert_outputs)
  VCU1 SCP/1(VACC_EACTempWarnInd_flg) -> [VACC_EACTempWarnInd_flg]
  VCU1 SCP/2(VACC_EACPressWarnInd_flg) -> [VACC_EACPressWarnInd_flg]
  [VACC_EACTempWarnInd_flg] -> Bus Creator/11
  [VACC_EACPressWarnInd_flg] -> Bus Creator/12
  [BSCP_In_outputs] -> AirPressure SCP/1(BSCP_In_outputs)
  AirPressure SCP/1(VACC_AirPressureFDisp_kpa) -> [VACC_AirPressureFDisp_kpa]
  AirPressure SCP/2(VACC_AirPressureRDisp_kpa) -> [VACC_AirPressureRDisp_kpa]
  AirPressure SCP/3(VACC_AirPressurePDisp_kpa) -> [VACC_AirPressurePDisp_kpa]
  [VACC_AirPressureFDisp_kpa] -> Bus Creator/13
  [VACC_AirPressureRDisp_kpa] -> Bus Creator/14
  [VACC_AirPressurePDisp_kpa] -> Bus Creator/15

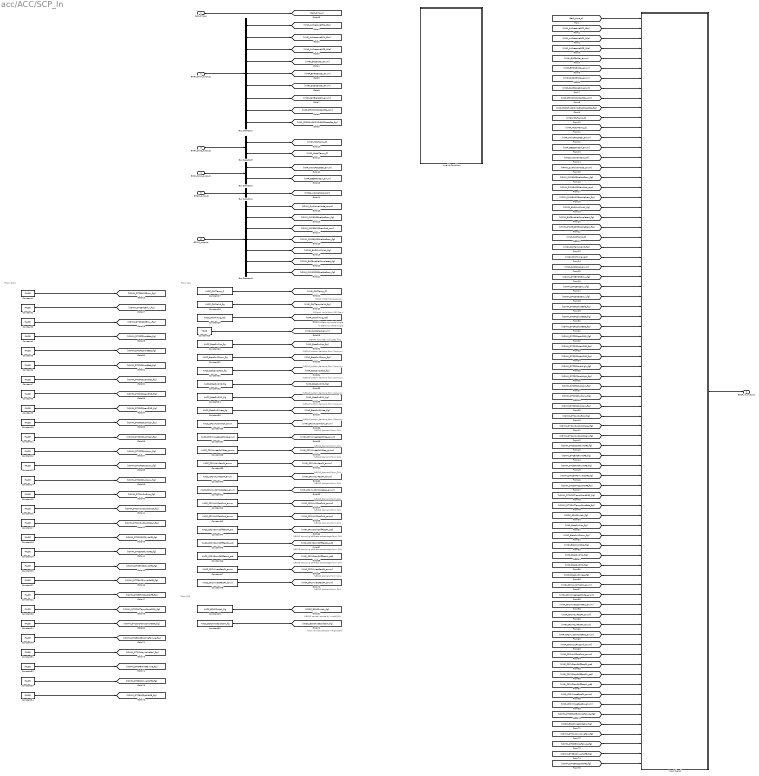
== system acc/ACC/SCP_In ==
  note: %ECAS demand form CAN.
  note: From DID
  note: FRom DDM
  note: From CAN
  note: %EAC Moter Temperature.
  note: %Signal valid from INP libary.
  note: %Steering wheel angle
  note: %EHPS has been adjusted flag.
  note: % Steering wheel angle
  note: %ECAS buttom demand form Zone pin.
  note: %ECAS buttom demand form Zone pin.
  note: %ECAS buttom demand form Zone pin.
  note: %ECAS buttom demand form Zone pin.
  note: %ECAS buttom demand form Zone pin.
  note: %ECAS buttom demand form Zone pin.
  note: %ECAS demand form CAN.
  note: %ECAS demand form CAN.
  note: %ECAS demand form CAN.
  note: %ECAS demand form CAN.
  note: %ECAS demand form CAN.
  note: %ECAS demand form CAN.
  note: %ECAS demand form CAN.
  note: %ECAS demand form CAN.
  note: %ECAS demand form CAN.
  note: %ECAS damping stiffness percentage form CAN.
  note: %ECAS damping stiffness percentage form CAN.
  note: %ECAS damping stiffness percentage form CAN.
  note: %ECAS control source by wired/CAN.
  note: %Driver side selection (Right/Left).
  task_time_s : Inport
  BINP_CAN4_outputs : Inport  Port=2
  BINP_CAN3_outputs : Inport  Port=3
  BINP_CAN1_outputs : Inport  Port=4
  BTQD_outputs : Inport  Port=5
  BPMM_outputs : Inport  Port=6
  Bus Selector1 : BusSelector  OutputSignals=VINP_AirPressureFC2_kPa,VINP_AirPressureRC1_kPa,VINP_AirPressurePC3_kPa,VINP_EACEnSta_enum,VINP_EHPSEnSta_enum,VINP_DCDCEnSta_enum,VINP_ParkBrakeSW_enum,VINP_EHPSMotorSpdSta_rpm,VINP_FDCCHASSISVCUEACPressSta_flg
  Bus Selector2 : BusSelector  OutputSignals=VINP_TransReqGear_enum,VINP_EBSBrakeSw_enum
  Bus Selector3 : BusSelector  OutputSignals=VINP_MCUTemp_C,VINP_MotorTemp_C
  Bus Selector4 : BusSelector  OutputSignals=VTQD_VCUVehSpd_kph
  Bus Selector6 : BusSelector  OutputSignals=VPMM_SysPowerMode_enum,VPMM_PMMEACEnableDem_flg,VPMM_PMMEHPSDemSpd_rpm,VPMM_PMMEHPSEnableDem_flg,VPMM_EHPSIniFinish_flg,VPMM_EACEnableCompleted_flg,VPMM_PMMDCDCEnableDem_flg
  Constant{1..24,49,51..54} (29 alike) : Constant  Value=FALSE
  Constant25 : Constant  Value=KACC_ECASSwitch_flg
  Constant26 : Constant  Value=KACC_CACValid_flg
  Constant27 : Constant  Value=KACC_CACTemp_C
  Constant28 : Constant  Value=KACC_StrWhlAng_rad
  Constant29 : Constant  Value=TRUE
  Constant30 : Constant  Value=KACC_EcasSw1Up_flg
  Constant31 : Constant  Value=KACC_EcasSw1Down_flg
  Constant32 : Constant  Value=KACC_EcasSw2Stop_flg
  Constant33 : Constant  Value=KACC_EcasSw2M2_flg
  Constant34 : Constant  Value=KACC_EcasSw3M1_flg
  Constant35 : Constant  Value=KACC_EcasSw3Knee_flg
  Constant36 : Constant  Value=KACC_CP2VAutoTracH_enum
  Constant37 : Constant  Value=KACC_CP2VKneeReqRSide_enum
  Constant38 : Constant  Value=KACC_CP2VKneeCtrlMReq_enum
  Constant39 : Constant  Value=KACC_CP2VNLvReqFA_enum
  Constant40 : Constant  Value=KACC_CP2VNLvReqRA_enum
  Constant41 : Constant  Value=KACC_CP2VLvCtrlModeReq_enum
  Constant42 : Constant  Value=KACC_CP2VLA1PosCmd_enum
  Constant43 : Constant  Value=KACC_CP2VLA2PosCmd_enum
  Constant44 : Constant  Value=KACC_CP2VDamStiffReqFA_pct
  Constant45 : Constant  Value=KACC_CP2VDamStiffReqRA_pct
  Constant46 : Constant  Value=KACC_CP2VDamStiffReqLA_pct
  Constant47 : Constant  Value=KACC_CP2VKneeReqFA_enum
  Constant48 : Constant  Value=KACC_CP2VKneeReqRA_enum
  Constant50 : Constant  Value=KACC_ECASKneeSideSW_flg
  Input Signal : Subsystem
  Invalid Condition : Subsystem
      settings: RTWSystemCode=Nonreusable function
  BSCP_In_outputs : Outport
  wires:
  Bus Selector4/1 -> [VTQD_VCUVehSpd_kph]  "<VTQD_VCUVehSpd_kph>"
  Bus Selector6/2 -> [VPMM_PMMEACEnableDem_flg]  "<VPMM_PMMEACEnableDem_flg>"
  Bus Selector6/3 -> [VPMM_PMMEHPSDemSpd_rpm]  "<VPMM_PMMEHPSDemSpd_rpm>"
  Bus Selector6/1 -> [VPMM_SysPowerMode_enum]  "<VPMM_SysPowerMode_enum>"
  Bus Selector1/7 -> [VINP_ParkBrakeSW_enum]  "<VINP_ParkBrakeSW_enum>"
  Bus Selector6/5 -> [VPMM_EHPSIniFinish_flg]  "<VPMM_EHPSIniFinish_flg>"
  BTQD_outputs/1 -> Bus Selector4/1
  Bus Selector6/4 -> [VPMM_PMMEHPSEnableDem_flg]  "<VPMM_PMMEHPSEnableDem_flg>"
  Bus Selector1/9 -> [VINP_FDCCHASSISVCUEACPressSta_flg]  "<VINP_FDCCHASSISVCUEACPressSta_flg>"
  Bus Selector6/7 -> [VPMM_PMMDCDCEnableDem_flg]  "<VPMM_PMMDCDCEnableDem_flg>"
  Bus Selector1/2 -> [VINP_AirPressureRC1_kPa]  "<VINP_AirPressureRC1_kPa>"
  Bus Selector6/6 -> [VPMM_EACEnableCompleted_flg]  "<VPMM_EACEnableCompleted_flg>"
  BPMM_outputs/1 -> Bus Selector6/1
  Bus Selector1/5 -> [VINP_EHPSEnSta_enum]  "<VINP_EHPSEnSta_enum>"
  Bus Selector3/1 -> [VINP_MCUTemp_C]  "<VINP_MCUTemp_C>"
  Bus Selector3/2 -> [VINP_MotorTemp_C]  "<VINP_MotorTemp_C>"
  BINP_CAN4_outputs/1 -> Bus Selector1/1
  Bus Selector1/3 -> [VINP_AirPressurePC3_kPa]  "<VINP_AirPressurePC3_kPa>"
  Bus Selector1/6 -> [VINP_DCDCEnSta_enum]  "<VINP_DCDCEnSta_enum>"
  Bus Selector1/4 -> [VINP_EACEnSta_enum]  "<VINP_EACEnSta_enum>"
  Bus Selector1/8 -> [VINP_EHPSMotorSpdSta_rpm]  "<VINP_EHPSMotorSpdSta_rpm>"
  Bus Selector2/1 -> [VINP_TransReqGear_enum]  "<VINP_TransReqGear_enum>"
  Bus Selector2/2 -> [VINP_EBSBrakeSw_enum]  "<VINP_EBSBrakeSw_enum>"
  Bus Selector1/1 -> [VINP_AirPressureFC2_kPa]  "<VINP_AirPressureFC2_kPa>"
  BINP_CAN3_outputs/1 -> Bus Selector3/1
  BINP_CAN1_outputs/1 -> Bus Selector2/1
  task_time_s/1 -> [task_time_s]
  Constant27/1 -> [VINP_CACTemp_C]
  Constant26/1 -> [VINP_CACTempValid_flg]
  Constant28/1 -> [VINP_StrWhlAng_rad]
  Constant29/1 -> [VINP_SASCaled_enum]
  Constant1/1 -> [VDMM_DTCEHPSErrLv_flg]
  Constant2/1 -> [VDMM_DTCEACErrLv_flg]
  Constant4/1 -> [VDMM_DTCFCShortBatt_flg]
  Constant3/1 -> [VDMM_DTCDCDCErrLv_flg]
  Constant7/1 -> [VDMM_DTCFCOpenGND_flg]
  Constant8/1 -> [VDMM_DTCPCOpenGND_flg]
  Constant6/1 -> [VDMM_DTCRCShortBatt_flg]
  Constant5/1 -> [VDMM_DTCPCShortBatt_flg]
  Constant13/1 -> [VDMM_DTCPCStuckLow_flg]
  Constant14/1 -> [VDMM_DTCRCStuckLow_flg]
  Constant16/1 -> [VDMM_DTCAirSwStuckClose_flg]
  Constant15/1 -> [VDMM_DTCAirSwError_flg]
  Constant11/1 -> [VDMM_DTCRCStuckHigh_flg]
  Constant12/1 -> [VDMM_DTCFCStuckLow_flg]
  Constant10/1 -> [VDMM_DTCFCStuckHigh_flg]
  Constant9/1 -> [VDMM_DTCRCOpenGND_flg]
  Constant17/1 -> [VDMM_DTCAirSwStuckOpen_flg]
  Constant19/1 -> [VDMM_DTCEACRlyNoFB_flg]
  Constant18/1 -> [VDMM_DTCDCDCRlyNoFB_flg]
  Constant20/1 -> [VDMM_DTCEHPSRlyNoFB_flg]
  Constant21/1 -> [VDMM_DTCEHPSInverNoFB_flg]
  Constant22/1 -> [VDMM_DTCEHPSSpdNoFB_flg]
  [task_time_s] -> Input Signal/1(task_time_s)
  [VINP_AirPressureFC2_kPa] -> Input Signal/2(VINP_AirPressureFC2_kPa)
  [VINP_AirPressureRC1_kPa] -> Input Signal/3(VINP_AirPressureRC1_kPa)
  [VINP_AirPressurePC3_kPa] -> Input Signal/4(VINP_AirPressurePC3_kPa)
  [VINP_EACEnSta_enum] -> Input Signal/5(VINP_EACEnSta_enum)
  [VINP_EHPSEnSta_enum] -> Input Signal/6(VINP_EHPSEnSta_enum)
  [VINP_DCDCEnSta_enum] -> Input Signal/7(VINP_DCDCEnSta_enum)
  [VINP_ParkBrakeSW_enum] -> Input Signal/8(VINP_ParkBrakeSW_enum)
  [VINP_EHPSMotorSpdSta_rpm] -> Input Signal/9(VINP_EHPSMotorSpdSta_rpm)
  [VINP_FDCCHASSISVCUEACPressSta_flg] -> Input Signal/10(VINP_FDCCHASSISVCUEACPressSta_flg)
  [VINP_MCUTemp_C] -> Input Signal/11(VINP_MCUTemp_C)
  [VINP_MotorTemp_C] -> Input Signal/12(VINP_MotorTemp_C)
  [VINP_TransReqGear_enum] -> Input Signal/13(VINP_TransReqGear_enum)
  [VINP_EBSBrakeSw_enum] -> Input Signal/14(VINP_EBSBrakeSw_enum)
  [VTQD_VCUVehSpd_kph] -> Input Signal/15(VTQD_VCUVehSpd_kph)
  [VPMM_SysPowerMode_enum] -> Input Signal/16(VPMM_SysPowerMode_enum)
  [VPMM_PMMEACEnableDem_flg] -> Input Signal/17(VPMM_PMMEACEnableDem_flg)
  [VPMM_PMMEHPSDemSpd_rpm] -> Input Signal/18(VPMM_PMMEHPSDemSpd_rpm)
  [VPMM_PMMEHPSEnableDem_flg] -> Input Signal/19(VPMM_PMMEHPSEnableDem_flg)
  [VPMM_EHPSIniFinish_flg] -> Input Signal/20(VPMM_EHPSIniFinish_flg)
  [VPMM_EACEnableCompleted_flg] -> Input Signal/21(VPMM_EACEnableCompleted_flg)
  [VPMM_PMMDCDCEnableDem_flg] -> Input Signal/22(VPMM_PMMDCDCEnableDem_flg)
  [VINP_CACTemp_C] -> Input Signal/23(VINP_CACTemp_C)
  [VINP_CACTempValid_flg] -> Input Signal/24(VINP_CACTempValid_flg)
  [VINP_StrWhlAng_rad] -> Input Signal/25(VINP_StrWhlAng_rad)
  [VINP_SASCaled_enum] -> Input Signal/26(VINP_SASCaled_enum)
  [VDMM_DTCEHPSErrLv_flg] -> Input Signal/27(VDMM_DTCEHPSErrLv_flg)
  [VDMM_DTCEACErrLv_flg] -> Input Signal/28(VDMM_DTCEACErrLv_flg)
  [VDMM_DTCDCDCErrLv_flg] -> Input Signal/29(VDMM_DTCDCDCErrLv_flg)
  [VDMM_DTCFCShortBatt_flg] -> Input Signal/30(VDMM_DTCFCShortBatt_flg)
  [VDMM_DTCPCShortBatt_flg] -> Input Signal/31(VDMM_DTCPCShortBatt_flg)
  [VDMM_DTCRCShortBatt_flg] -> Input Signal/32(VDMM_DTCRCShortBatt_flg)
  [VDMM_DTCFCOpenGND_flg] -> Input Signal/33(VDMM_DTCFCOpenGND_flg)
  [VDMM_DTCPCOpenGND_flg] -> Input Signal/34(VDMM_DTCPCOpenGND_flg)
  [VDMM_DTCRCOpenGND_flg] -> Input Signal/35(VDMM_DTCRCOpenGND_flg)
  [VDMM_DTCFCStuckHigh_flg] -> Input Signal/36(VDMM_DTCFCStuckHigh_flg)
  [VDMM_DTCRCStuckHigh_flg] -> Input Signal/37(VDMM_DTCRCStuckHigh_flg)
  [VDMM_DTCFCStuckLow_flg] -> Input Signal/38(VDMM_DTCFCStuckLow_flg)
  [VDMM_DTCPCStuckLow_flg] -> Input Signal/39(VDMM_DTCPCStuckLow_flg)
  [VDMM_DTCRCStuckLow_flg] -> Input Signal/40(VDMM_DTCRCStuckLow_flg)
  [VDMM_DTCAirSwError_flg] -> Input Signal/41(VDMM_DTCAirSwError_flg)
  [VDMM_DTCAirSwStuckClose_flg] -> Input Signal/42(VDMM_DTCAirSwStuckClose_flg)
  [VDMM_DTCAirSwStuckOpen_flg] -> Input Signal/43(VDMM_DTCAirSwStuckOpen_flg)
  [VDMM_DTCDCDCRlyNoFB_flg] -> Input Signal/44(VDMM_DTCDCDCRlyNoFB_flg)
  [VDMM_DTCEACRlyNoFB_flg] -> Input Signal/45(VDMM_DTCEACRlyNoFB_flg)
  [VDMM_DTCEHPSRlyNoFB_flg] -> Input Signal/46(VDMM_DTCEHPSRlyNoFB_flg)
  [VDMM_DTCEHPSInverNoFB_flg] -> Input Signal/47(VDMM_DTCEHPSInverNoFB_flg)
  [VDMM_DTCEHPSSpdNoFB_flg] -> Input Signal/48(VDMM_DTCEHPSSpdNoFB_flg)
  Input Signal/1(BSCP_In_outputs) -> BSCP_In_outputs/1
  Constant24/1 -> [VDMM_DTCCACTempShortBatt_flg]
  Constant23/1 -> [VDMM_DTCCACTempShortGND_flg]
  [VDMM_DTCCACTempShortGND_flg] -> Input Signal/49(VDMM_DTCCACTempShortGND_flg)
  [VDMM_DTCCACTempShortBatt_flg] -> Input Signal/50(VDMM_DTCCACTempShortBatt_flg)
  Constant25/1 -> [VDSC_ECASSwitch_flg]
  Constant30/1 -> [VINP_EcasSw1Up_flg]
  Constant31/1 -> [VINP_EcasSw1Down_flg]
  Constant32/1 -> [VINP_EcasSw2Stop_flg]
  Constant33/1 -> [VINP_EcasSw2M2_flg]
  [VDSC_ECASSwitch_flg] -> Input Signal/51(VDSC_ECASSwitch_flg)
  Constant34/1 -> [VINP_EcasSw3M1_flg]
  Constant35/1 -> [VINP_EcasSw3Knee_flg]
  [VINP_EcasSw1Up_flg] -> Input Signal/52(VINP_EcasSw1Up_flg)
  [VINP_EcasSw1Down_flg] -> Input Signal/53(VINP_EcasSw1Down_flg)
  [VINP_EcasSw2Stop_flg] -> Input Signal/54(VINP_EcasSw2Stop_flg)
  [VINP_EcasSw2M2_flg] -> Input Signal/55(VINP_EcasSw2M2_flg)
  [VINP_EcasSw3M1_flg] -> Input Signal/56(VINP_EcasSw3M1_flg)
  [VINP_EcasSw3Knee_flg] -> Input Signal/57(VINP_EcasSw3Knee_flg)
  Constant36/1 -> [VINP_CP2VAutoTracH_enum]
  Constant37/1 -> [VINP_CP2VKneeReqRSide_enum]
  Constant38/1 -> [VINP_CP2VKneeCtrlMReq_enum]
  Constant39/1 -> [VINP_CP2VNLvReqFA_enum]
  Constant40/1 -> [VINP_CP2VNLvReqRA_enum]
  Constant41/1 -> [VINP_CP2VLvCtrlModeReq_enum]
  Constant42/1 -> [VINP_CP2VLA1PosCmd_enum]
  Constant43/1 -> [VINP_CP2VLA2PosCmd_enum]
  Constant44/1 -> [VINP_CP2VDamStiffReqFA_pct]
  Constant45/1 -> [VINP_CP2VDamStiffReqRA_pct]
  Constant46/1 -> [VINP_CP2VDamStiffReqLA_pct]
  Constant47/1 -> [VINP_CP2VKneeReqFA_enum]
  Constant48/1 -> [VINP_CP2VKneeReqRA_enum]
  Constant49/1 -> [VDMM_DTCECASButWireFailure_flg]
  [VINP_CP2VAutoTracH_enum] -> Input Signal/58(VINP_CP2VAutoTracH_enum)
  [VINP_CP2VKneeReqRSide_enum] -> Input Signal/59(VINP_CP2VKneeReqRSide_enum)
  [VINP_CP2VKneeCtrlMReq_enum] -> Input Signal/60(VINP_CP2VKneeCtrlMReq_enum)
  [VINP_CP2VNLvReqFA_enum] -> Input Signal/61(VINP_CP2VNLvReqFA_enum)
  [VINP_CP2VNLvReqRA_enum] -> Input Signal/62(VINP_CP2VNLvReqRA_enum)
  [VINP_CP2VLvCtrlModeReq_enum] -> Input Signal/63(VINP_CP2VLvCtrlModeReq_enum)
  [VINP_CP2VLA1PosCmd_enum] -> Input Signal/64(VINP_CP2VLA1PosCmd_enum)
  [VINP_CP2VLA2PosCmd_enum] -> Input Signal/65(VINP_CP2VLA2PosCmd_enum)
  [VINP_CP2VDamStiffReqFA_pct] -> Input Signal/66(VINP_CP2VDamStiffReqFA_pct)
  [VINP_CP2VDamStiffReqRA_pct] -> Input Signal/67(VINP_CP2VDamStiffReqRA_pct)
  [VINP_CP2VDamStiffReqLA_pct] -> Input Signal/68(VINP_CP2VDamStiffReqLA_pct)
  [VINP_CP2VKneeReqFA_enum] -> Input Signal/69(VINP_CP2VKneeReqFA_enum)
  [VINP_CP2VKneeReqRA_enum] -> Input Signal/70(VINP_CP2VKneeReqRA_enum)
  [VDMM_DTCECASButWireFailure_flg] -> Input Signal/71(VDMM_DTCECASButWireFailure_flg)
  Constant50/1 -> [VDSC_ECASKneeSideSW_flg]
  [VDSC_ECASKneeSideSW_flg] -> Input Signal/72(VDSC_ECASKneeSideSW_flg)
  Constant51/1 -> [VDMM_DTC4WayValveFail_flg]
  Constant52/1 -> [VDMM_DTCPBWireFailure_flg]
  Constant53/1 -> [VDMM_DTCEACInverNoFB_flg]
  Constant54/1 -> [VDMM_DTCEACSpdNoFB_flg]
  [VDMM_DTC4WayValveFail_flg] -> Input Signal/73(VDMM_DTC4WayValveFail_flg)
  [VDMM_DTCPBWireFailure_flg] -> Input Signal/74(VDMM_DTCPBWireFailure_flg)
  [VDMM_DTCEACInverNoFB_flg] -> Input Signal/75(VDMM_DTCEACInverNoFB_flg)
  [VDMM_DTCEACSpdNoFB_flg] -> Input Signal/76(VDMM_DTCEACSpdNoFB_flg)
